simulink model "proiectFCO"  (R2020b)
settings: Solver=VariableStepAuto  StartTime=0.0  StopTime=10  RelTol=1e-3
values from neighbouring files (symbols this model uses):
  A = [0 0 1 0 ... (first row only)    [proiectTS.m]
  a0 = den(5)    [proiectTS.m]
  a1 = den(4)    [proiectTS.m]
  a2 = den(3)    [proiectTS.m]
  a3 = den(2)    [proiectTS.m]
  B = [0 0 1/m1 0]'    [proiectTS.m]
  b10 = num(1,5)    [proiectTS.m]
  b11 = num(1,4)    [proiectTS.m]
  b12 = num(1,3)    [proiectTS.m]
  C = [1 0 0 0 ... (first row only)    [proiectTS.m]
  D = [0 0]'    [proiectTS.m]
undefined symbols (not defined in the file or in its folder): den, num
settings Model: Creator=Alex  LastModifiedBy=Alex

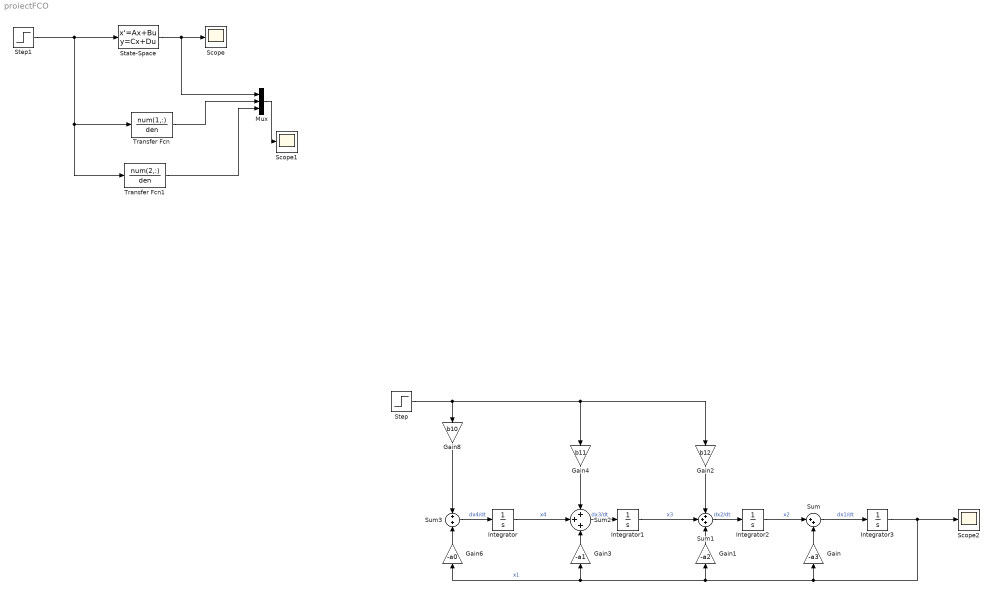
== system proiectFCO ==
  Gain : Gain  Gain=-a3
  Gain1 : Gain  Gain=-a2
  Gain2 : Gain  Gain=b12
  Gain3 : Gain  Gain=-a1
  Gain4 : Gain  Gain=b11
  Gain6 : Gain  Gain=-a0
  Gain8 : Gain  Gain=b10
  Integrator{,1..3} (4 alike) : Integrator
  Mux : Mux  Inputs=3
  Scope : Scope
  Scope1 : Scope
  Scope2 : Scope
  State-Space : StateSpace  A=A  B=B  C=C  D=D  InitialCondition=0
  Step : Step  SampleTime=0
  Step1 : Step  SampleTime=0
  Sum : Sum  Inputs=|++
  Sum1 : Sum  Inputs=+++
  Sum2 : Sum  Inputs=+++
  Sum3 : Sum
  Transfer Fcn : TransferFcn  Numerator=num(1,:)  Denominator=den
  Transfer Fcn1 : TransferFcn  Numerator=num(2,:)  Denominator=den
  wires:
  State-Space/1 -> Mux/1, Scope/1
  Step1/1 -> Transfer Fcn1/1, Transfer Fcn/1, State-Space/1
  Mux/1 -> Scope1/1
  Transfer Fcn1/1 -> Mux/3
  Transfer Fcn/1 -> Mux/2
  Integrator3/1 -> Scope2/1, Gain6/1, Gain3/1, Gain1/1, Gain/1  "x1"
  Integrator2/1 -> Sum/1  "x2"
  Sum/1 -> Integrator3/1  "dx1/dt"
  Gain/1 -> Sum/2
  Gain1/1 -> Sum1/3
  Integrator1/1 -> Sum1/2  "x3"
  Sum1/1 -> Integrator2/1  "dx2/dt"
  Gain2/1 -> Sum1/1
  Sum2/1 -> Integrator1/1  "dx3/dt"
  Gain3/1 -> Sum2/3
  Step/1 -> Gain4/1, Gain2/1, Gain8/1
  Gain4/1 -> Sum2/1
  Sum3/1 -> Integrator/1  "dx4/dt"
  Gain6/1 -> Sum3/2
  Gain8/1 -> Sum3/1
  Integrator/1 -> Sum2/2  "x4"
